simulink model "power_3phmutseq10"  (Simulink 6.0)
settings: Solver=ode23tb  StartTime=0.0  StopTime=0.2  RelTol=1e-4
libraries: powerlib x6, powerlib_extras x1
settings Model: Creator=by2815  LastModifiedBy=batserve  ExtModeAutoUpdateStatusClock=off
settings DataIOCC: SaveOutput=off  SaveTime=off  SignalLoggingName=sigsOut
settings DebuggingCC: SolverPrmCheckMsg=none
settings HardwareCC: TargetUnknown=on

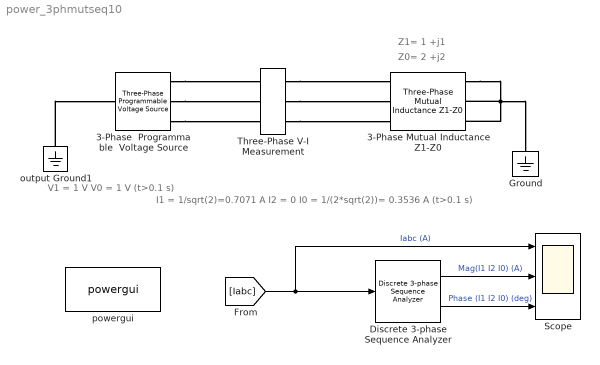
== system power_3phmutseq10 ==
  note: V1 = 1 V
      | V0 = 1 V (t>0.1 s)
  note: Z1= 1 +j1
  note: Z0= 2 +j2
  note: I1 = 1/sqrt(2)=0.7071 A
      | I2 = 0
      | I0 = 1/(2*sqrt(2))= 0.3536 A (t>0.1 s)
  3-Phase Mutual Inductance Z1-Z0 : powerlib/Elements/Three-Phase Mutual Inductance Z1-Z0  PhysicalDomain=powersysdomain  SubClassName=unknown  LeftPortType=p1  RightPortType=p1  LConnTagsString=a|b|c  RConnTagsString=A|B|C  PositiveSequence=[ 1 1/(2*pi*60)]  ZeroSequence=[1 1/(2*pi*60)]*2
  3-Phase  Programmable  Voltage Source : powerlib/Electrical Sources/Three-Phase Programmable Voltage Source  PositiveSequence="[1/sqrt(2)*sqrt(3) 0  60]"  VariationEntity=None  VariationType=Modulation  VariationStep=-0.3  VariationRate=0.5  VariationMagnitude=0.4  VariationFrequency=2  VariationTiming=[0.1 1.2]  VariationPhaseA=off  Amplitudes="[1  0.8  1.2  1.0 ]"  TimeValues=[0 0.1 0.25 0.4]  HarmonicGeneration=on  HarmonicA=[1 1 0 0]  HarmonicB="[2 0.0  0  2]"  Timing="[0.1  10]"
  Discrete 3-phase Sequence Analyzer : powerlib_extras/Discrete Measurements/Discrete 3-phase Sequence Analyzer  Freq=60  n=1  seq=Positive Negative Zero  Par_Init=[0 0]  Ts=50e-6
  Ground : powerlib/Elements/Ground  Orientation=down  PhysicalDomain=powersysdomain  SubClassName=unknown  LeftPortType=p1  RightPortType=p1  LConnTagsString=a
  Scope : Scope  NumInputPorts=3
      settings: TimeRange=0.2  YMin=-2~0~-50  YMax=2~0.8~100
  Three-Phase V-I Measurement : powerlib/Measurements/Three-Phase V-I Measurement  VoltageMeasurement=no  SetLabelV=off  LabelV=Vabc  Vpu=off  Vbase=500e3  CurrentMeasurement=yes  SetLabelI=on  LabelI=Iabc  Ipu=off  Pbase=100e6  OutputType=Magnitude  PhasorSimulation=off  PSBequivalent=0
  output Ground1 : powerlib/Elements/Ground  Orientation=down  PhysicalDomain=powersysdomain  SubClassName=unknown  LeftPortType=p1  RightPortType=p1  LConnTagsString=a
  powergui : powerlib/powergui  Priority=2  Frange=[0:2:500]  Ylog=off  Xlog=off  save=off  variable=ZData  ZoomFFT=on  StartTime=0.0  cycles=1  DisplayStyle=off  fundamental=60  FreqAxis=off  MaxFrequency=1000  frequencyindice=1  frequencyindicesteady=1  RmsSteady=1  display=off  Ts=50e-6  methode=off  frequency=60  echomessages=off
  wires:
  Discrete 3-phase Sequence Analyzer/1 -> Scope/2  "Mag(I1 I2 I0) (A)"
  [Iabc] -> Discrete 3-phase Sequence Analyzer/1, Scope/1  "Iabc (A)"
  Discrete 3-phase Sequence Analyzer/2 -> Scope/3  "Phase (I1 I2 I0) (deg)"
  connections:
  output Ground1/LConn1 -- 3-Phase  Programmable  Voltage Source/LConn1
  3-Phase Mutual Inductance Z1-Z0/RConn1 -- 3-Phase Mutual Inductance Z1-Z0/RConn2 -- 3-Phase Mutual Inductance Z1-Z0/RConn3 -- Ground/LConn1
  Three-Phase V-I Measurement/RConn1 -- 3-Phase Mutual Inductance Z1-Z0/LConn1
  Three-Phase V-I Measurement/RConn2 -- 3-Phase Mutual Inductance Z1-Z0/LConn2
  Three-Phase V-I Measurement/RConn3 -- 3-Phase Mutual Inductance Z1-Z0/LConn3
  3-Phase  Programmable  Voltage Source/RConn1 -- Three-Phase V-I Measurement/LConn1
  3-Phase  Programmable  Voltage Source/RConn2 -- Three-Phase V-I Measurement/LConn2
  3-Phase  Programmable  Voltage Source/RConn3 -- Three-Phase V-I Measurement/LConn3
